simulink model "s_diff2"  (Simulink 4.00)
settings: Solver=ode5  SolverMode=SingleTasking  StartTime=0.0  StopTime=3e-4  FixedStep=1e-7  MaxStep=1e-7  RelTol=1e-3  AbsTol=1e-6
libraries: simulink3 x1
settings Model: LastModifiedBy=Administrator  SaveTime=off  SaveOutput=off  LimitDataPoints=off  BlockReductionOpt=off

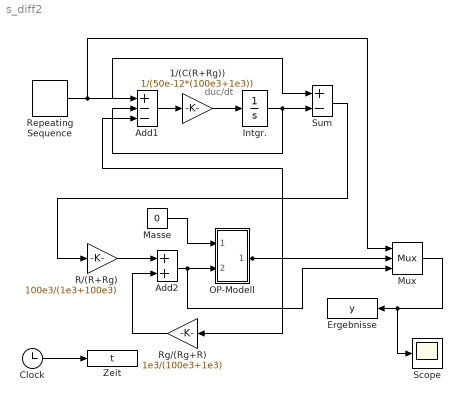
== system s_diff2 ==
  note: duc/dt
  1/(C(R+Rg)) : Gain  Gain=1/(50e-12*(100e3+1e3))  Multiplication=Element-wise(K.*u)  SaturateOnIntegerOverflow=on
  Add1 : Sum  Inputs=+--  SaturateOnIntegerOverflow=on
  Add2 : Sum  Inputs=++  SaturateOnIntegerOverflow=on
  Clock : Clock
      settings: DisplayTime=off  Decimation=10
  Ergebnisse : ToWorkspace  VariableName=y  SampleTime=0  SaveFormat=Array
      settings: MaxDataPoints=1000
  Intgr. : Integrator  ExternalReset=none  InitialConditionSource=internal  InitialCondition=0  LimitOutput=off  UpperSaturationLimit=inf  LowerSaturationLimit=-inf  ShowSaturationPort=off  ShowStatePort=off  AbsoluteTolerance=auto
  Masse : Constant  Value=0
  Mux : Mux  Inputs=3
      settings: DisplayOption=none
  OP-Modell : Subsystem
      settings: RTWFcnNameOpts=Auto  RTWFileNameOpts=Auto
  R/(R+Rg) : Gain  Gain=100e3/(1e3+100e3)  Multiplication=Element-wise(K.*u)  SaturateOnIntegerOverflow=on
  Repeating Sequence : simulink3/Sources/Repeating Sequence  rep_seq_t=[0, 10e-6, 20e-6, 30e-6, 40e-6]  rep_seq_y="[0 4  0 -4 0]"
  Rg/(Rg+R) : Gain  Orientation=left  Gain=1e3/(100e3+1e3)  Multiplication=Element-wise(K.*u)  SaturateOnIntegerOverflow=on
  Scope : Scope
      settings: TickLabels=on  TimeRange=0.0003  YMin=-7.4704  YMax=7.4704  SaveToWorkspace=off  SaveName=ScopeData  DataFormat=Array  LimitDataPoints=on  MaxDataPoints=5000
  Sum : Sum  Inputs=+-  SaturateOnIntegerOverflow=on
  Zeit : ToWorkspace  VariableName=t  SampleTime=0  SaveFormat=Array
      settings: MaxDataPoints=1000
  wires:
  Mux/1 -> Scope/1, Ergebnisse/1
  Clock/1 -> Zeit/1
  Add2/1 -> Mux/3, OP-Modell/2(in_2)
  Sum/1 -> R/(R+Rg)/1
  Rg/(Rg+R)/1 -> Add2/2
  R/(R+Rg)/1 -> Add2/1
  OP-Modell/1(out_1) -> Rg/(Rg+R)/1, Mux/2, Add1/3
  Intgr./1 -> Add1/2, Sum/2
  Repeating Sequence/1 -> Mux/1, Add1/1, Sum/1
  Add1/1 -> 1/(C(R+Rg))/1
  1/(C(R+Rg))/1 -> Intgr./1
  Masse/1 -> OP-Modell/1(in_1)

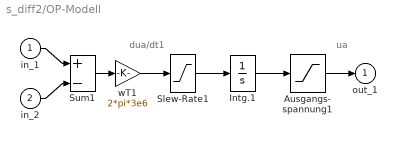
== system s_diff2/OP-Modell ==
  note: ua
  note: dua/dt1
  in_1 : Inport  Port=1
  in_2 : Inport  Port=2
  " wT1" : Gain  Gain=2*pi*3e6  Multiplication=Element-wise(K.*u)  SaturateOnIntegerOverflow=on
  Ausgangs- spannung1 : Saturate  UpperLimit=10  LowerLimit=-10  LinearizeAsGain=on
  Intg.1 : Integrator  ExternalReset=none  InitialConditionSource=internal  InitialCondition=0  LimitOutput=off  UpperSaturationLimit=inf  LowerSaturationLimit=-inf  ShowSaturationPort=off  ShowStatePort=off  AbsoluteTolerance=auto
  Slew-Rate1 : Saturate  UpperLimit=10e6  LowerLimit=-10e6  LinearizeAsGain=on
  Sum1 : Sum  Inputs=+-  SaturateOnIntegerOverflow=on
  out_1 : Outport  Port=1
  wires:
  Intg.1/1 -> Ausgangs- spannung1/1
  Slew-Rate1/1 -> Intg.1/1
  " wT1"/1 -> Slew-Rate1/1
  Sum1/1 -> " wT1"/1
  in_1/1 -> Sum1/1
  Ausgangs- spannung1/1 -> out_1/1
  in_2/1 -> Sum1/2
